simulink model "send_a825_r2019b"  (R2019b)
settings: Solver=VariableStepAuto  StartTime=0.0  StopTime=10.0  RelTol=1e-3
libraries: lib_ed247 x2
settings Model: Creator=odufour  LastModifiedBy=odufour

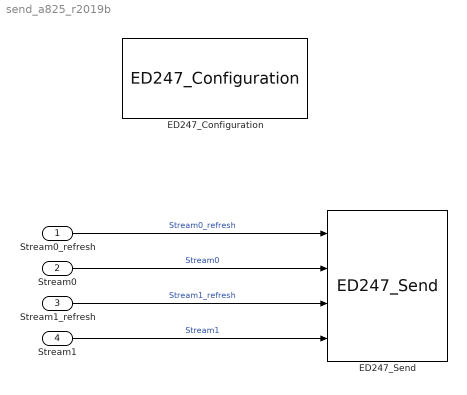
== system send_a825_r2019b ==
  Stream0_refresh : Inport  OutDataTypeStr=boolean  PortDimensions=1
  Stream0 : Inport  Port=2  OutDataTypeStr=uint8  PortDimensions=3  SampleTime=0.1
  Stream1_refresh : Inport  Port=3  OutDataTypeStr=boolean  PortDimensions=1
  Stream1 : Inport  Port=4  OutDataTypeStr=uint8  PortDimensions=5  SampleTime=0.1
  ED247_Configuration : lib_ed247/ED247_Configuration  configurationFilename='ecic_func_exchange_a825_uc_main.xml'  enableLog=off  logFilename='<PROJECT_FOLDER>\work\tmp.log'
      settings: SourceProductName=Airbus ED247
  ED247_Send : lib_ed247/ED247_Send  Parameter1=0
      settings: SourceProductName=Airbus ED247
  wires:
  Stream0/1 -> ED247_Send/2  "Stream0"
  Stream0_refresh/1 -> ED247_Send/1  "Stream0_refresh"
  Stream1_refresh/1 -> ED247_Send/3  "Stream1_refresh"
  Stream1/1 -> ED247_Send/4  "Stream1"
